simulink model "TotLabs_DCM"  (R2024b)
settings: Solver=VariableStepAuto  StartTime=0.0  StopTime=10.0  RelTol=1e-3
values from neighbouring files (symbols this model uses):
  Ar = [6e-2; 6e-2; 6e-2; 6e-2; 4e-2; 4e-2; 12e-2; 12e-2; 12e-2; 12e-2]    [LabsDCM.m]    (also in Srp_Lab7.m; airdrag.m)
  c = astroConstants(5)    [LabsDCM.m]    (also in Srp_Lab7.m; airdrag.m)
  Ep = deg2rad(epsilon)    [LabsDCM.m]    (also in Srp_Lab7.m = deg2rad(23.45); airdrag.m)
  Fe = 1358    [LabsDCM.m]    (also in airdrag.m)
  J = diag([Ix Iy Iz])    [LabsDCM.m]    (also in Srp_Lab7.m; airdrag.m)
  n = sqrt(G*M/(R^3))    [LabsDCM.m]    (also in Srp_Lab7.m; airdrag.m)
  N_B = [ 1,  0,  0 ... (first row only)    [LabsDCM.m]    (also in Srp_Lab7.m; airdrag.m)
  nx = 2*pi()/T    [LabsDCM.m]    (also in Srp_Lab7.m; airdrag.m)
  r_Fi = [ ... (first row only)    [LabsDCM.m]    (also in Srp_Lab7.m; airdrag.m)
  r_sun = astroConstants(2)    [LabsDCM.m]    (also in Srp_Lab7.m; airdrag.m = astroConstants(3))
  rho_d = [0.1; 0.1; 0.1; 0.1; 0.1; 0.1; 0.1; 0.1; 0.1; 0.1]    [LabsDCM.m]    (also in Srp_Lab7.m; airdrag.m)
  rho_s = [0.5; 0.5; 0.5; 0.5; 0.5; 0.5; 0.1; 0.1; 0.1; 0.1]    [LabsDCM.m]    (also in Srp_Lab7.m; airdrag.m)
  W0 = [0.45 0.52 0.55]    [LabsDCM.m]    (also in Srp_Lab7.m; airdrag.m)
libraries: matrix_library x3, vrlib x1
settings Model: Creator=User  LastModifiedBy=User

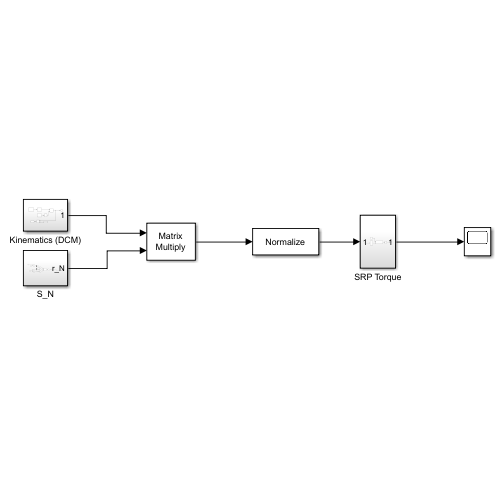
[thumbnail: Simulink's stored preview of the top-level diagram]
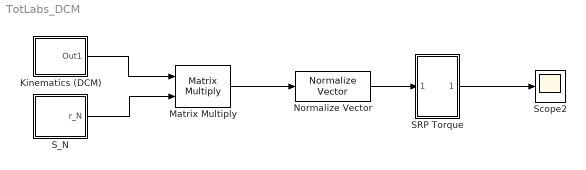
== system TotLabs_DCM ==
  Kinematics (DCM) : Subsystem
  Matrix Multiply : Product  Multiplication=Matrix(*)
  Normalize Vector : vrlib/Utilities/Normalize Vector  maxzero=0
  SRP Torque : Subsystem
  S_N : Subsystem
  Scope2 : Scope
  wires:
  Normalize Vector/1 -> SRP Torque/1(In1)
  SRP Torque/1(Out1) -> Scope2/1
  Matrix Multiply/1 -> Normalize Vector/1
  Kinematics (DCM)/1(Out1) -> Matrix Multiply/1
  S_N/1(r_N) -> Matrix Multiply/2

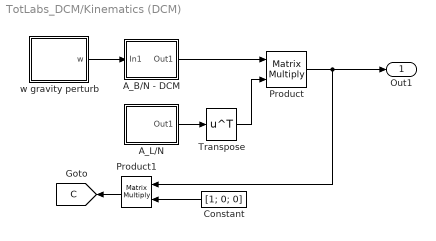
== system TotLabs_DCM/Kinematics (DCM) ==
  A_B/N - DCM : Subsystem
  A_L/N : Subsystem
  Constant : Constant  Value=[1; 0; 0]
  Product : Product  Multiplication=Matrix(*)
  Product1 : Product  Multiplication=Matrix(*)
  Transpose : Math  Operator=transpose
  w gravity perturb : Subsystem
  Out1 : Outport
  tag scope: C=global
  wires:
  A_L/N/1(Out1) -> Transpose/1
  Constant/1 -> Product1/2
  Product/1 -> Out1/1, Product1/1
  Transpose/1 -> Product/2
  A_B/N - DCM/1(Out1) -> Product/1
  Product1/1 -> [C]
  w gravity perturb/1(w) -> A_B/N - DCM/1(In1)

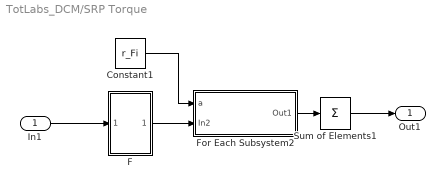
== system TotLabs_DCM/SRP Torque ==
  In1 : Inport
  Constant1 : Constant  Value=r_Fi
  F : Subsystem
  For Each Subsystem2 : Subsystem  TreatAsAtomicUnit=on
  Sum of Elements1 : Sum  Inputs=+  CollapseMode=Specified dimension
  Out1 : Outport
  wires:
  Constant1/1 -> For Each Subsystem2/1(a)
  For Each Subsystem2/1(Out1) -> Sum of Elements1/1
  Sum of Elements1/1 -> Out1/1
  In1/1 -> F/1(In1)
  F/1(Out1) -> For Each Subsystem2/2(In2)

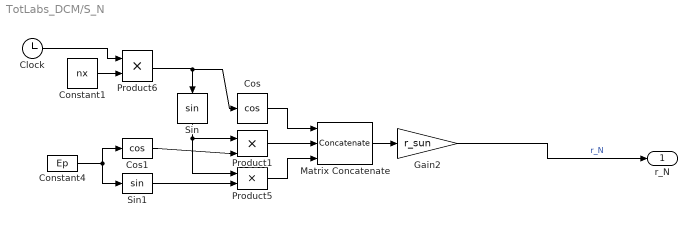
== system TotLabs_DCM/S_N ==
  Clock : Clock
  Constant1 : Constant  Value=nx
  Constant4 : Constant  Value=Ep
  Cos : Trigonometry  Operator=cos
  Cos1 : Trigonometry  Operator=cos
  Gain2 : Gain  Gain=r_sun
  Matrix Concatenate : Concatenate  NumInputs=3  Mode=Multidimensional array
  Product1 : Product
  Product5 : Product
  Product6 : Product
  Sin : Trigonometry
  Sin1 : Trigonometry
  r_N : Outport
  wires:
  Matrix Concatenate/1 -> Gain2/1
  Cos1/1 -> Product1/2
  Constant1/1 -> Product6/2
  Cos/1 -> Matrix Concatenate/1
  Product5/1 -> Matrix Concatenate/3
  Sin/1 -> Product5/1, Product1/1
  Clock/1 -> Product6/1
  Product1/1 -> Matrix Concatenate/2
  Sin1/1 -> Product5/2
  Product6/1 -> Cos/1, Sin/1
  Constant4/1 -> Sin1/1, Cos1/1
  Gain2/1 -> r_N/1  "r_N"

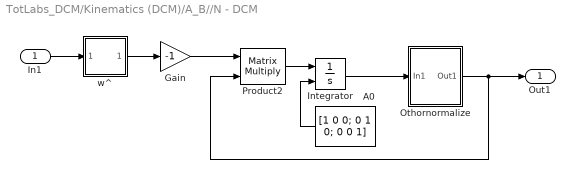
== system TotLabs_DCM/Kinematics (DCM)/A_B//N - DCM ==
  In1 : Inport
  A0 : Constant  Value=[1 0 0; 0 1 0; 0 0 1]
  Gain : Gain  Gain=-1
  Integrator : Integrator  InitialConditionSource=external
  Othornormalize : Subsystem
  Product2 : Product  Multiplication=Matrix(*)
  w^ : Subsystem
  Out1 : Outport
  wires:
  w^/1(Out1) -> Gain/1
  A0/1 -> Integrator/2
  Product2/1 -> Integrator/1
  In1/1 -> w^/1(In1)
  Othornormalize/1(Out1) -> Out1/1, Product2/2
  Integrator/1 -> Othornormalize/1(In1)
  Gain/1 -> Product2/1

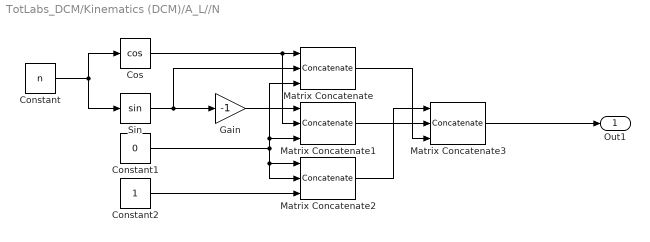
== system TotLabs_DCM/Kinematics (DCM)/A_L//N ==
  Constant : Constant  Value=n
  Constant1 : Constant  Value=0
  Constant2 : Constant
  Cos : Trigonometry  Operator=cos
  Gain : Gain  Gain=-1
  Matrix Concatenate : Concatenate  NumInputs=3  Mode=Multidimensional array
  Matrix Concatenate1 : Concatenate  NumInputs=3  Mode=Multidimensional array
  Matrix Concatenate2 : Concatenate  NumInputs=3  Mode=Multidimensional array
  Matrix Concatenate3 : Concatenate  NumInputs=3  Mode=Multidimensional array  ConcatenateDimension=2
  Sin : Trigonometry
  Out1 : Outport
  wires:
  Matrix Concatenate1/1 -> Matrix Concatenate3/2
  Matrix Concatenate3/1 -> Out1/1
  Constant1/1 -> Matrix Concatenate/3, Matrix Concatenate1/3, Matrix Concatenate2/2, Matrix Concatenate2/1
  Cos/1 -> Matrix Concatenate1/2, Matrix Concatenate/1
  Constant/1 -> Sin/1, Cos/1
  Constant2/1 -> Matrix Concatenate2/3
  Sin/1 -> Matrix Concatenate/2, Gain/1
  Gain/1 -> Matrix Concatenate1/1
  Matrix Concatenate2/1 -> Matrix Concatenate3/1
  Matrix Concatenate/1 -> Matrix Concatenate3/3

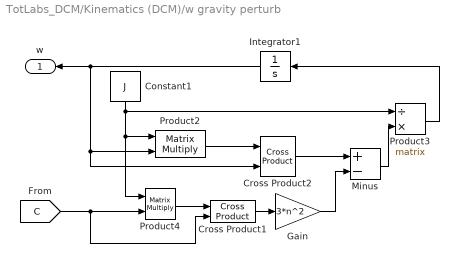
== system TotLabs_DCM/Kinematics (DCM)/w gravity perturb ==
  Constant1 : Constant  Value=J
  Cross Product1 : matrix_library/Cross Product
  Cross Product2 : matrix_library/Cross Product
  Gain : Gain  Gain=3*n^2
  Integrator1 : Integrator  InitialCondition=W0
  Minus : Sum  Inputs=+-
  Product2 : Product  Multiplication=Matrix(*)
  Product3 : Product  Inputs=/*  Multiplication=Matrix(*)
  Product4 : Product  Multiplication=Matrix(*)
  w : Outport
  wires:
  Integrator1/1 -> Cross Product2/2, Product2/2, w/1
  Minus/1 -> Product3/2
  Constant1/1 -> Product3/1, Product2/1, Product4/1
  Product3/1 -> Integrator1/1
  Product2/1 -> Cross Product2/1
  Cross Product2/1 -> Minus/1
  Cross Product1/1 -> Gain/1
  Gain/1 -> Minus/2
  Product4/1 -> Cross Product1/1
  [C] -> Product4/2, Cross Product1/2

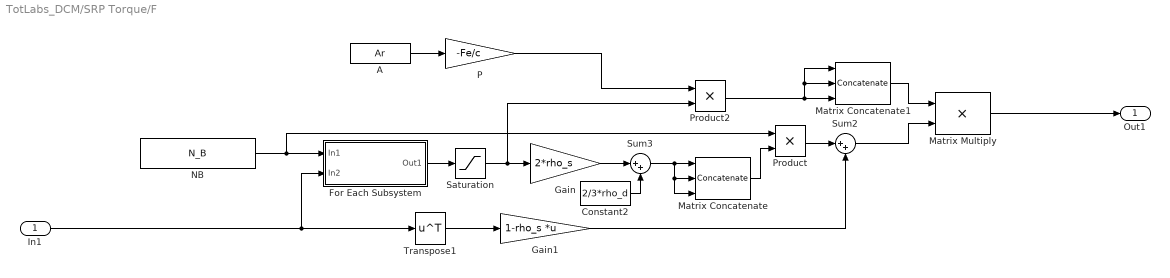
== system TotLabs_DCM/SRP Torque/F ==
  In1 : Inport
  A : Constant  Value=Ar
  Constant2 : Constant  Value=2/3*rho_d
  For Each Subsystem : Subsystem  TreatAsAtomicUnit=on
  Gain : Gain  Gain=2*rho_s
  Gain1 : Gain  Gain=1-rho_s  Multiplication=Matrix(K*u)
  Matrix Concatenate : Concatenate  NumInputs=3  Mode=Multidimensional array  ConcatenateDimension=2
  Matrix Concatenate1 : Concatenate  NumInputs=3  Mode=Multidimensional array  ConcatenateDimension=2
  Matrix Multiply : Product
  NB : Constant  Value=N_B
  P : Gain  Gain=-Fe/c
  Product : Product
  Product2 : Product
  Saturation : Saturate  UpperLimit=inf  LowerLimit=0
  Sum2 : Sum  Inputs=|++
  Sum3 : Sum  Inputs=|++
  Transpose1 : Math  Operator=transpose
  Out1 : Outport
  wires:
  For Each Subsystem/1(Out1) -> Saturation/1
  In1/1 -> For Each Subsystem/2(In2), Transpose1/1
  Matrix Concatenate/1 -> Product/2
  Gain/1 -> Sum3/1
  Saturation/1 -> Product2/2, Gain/1
  NB/1 -> For Each Subsystem/1(In1), Product/1
  Gain1/1 -> Sum2/2
  Matrix Concatenate1/1 -> Matrix Multiply/1
  Constant2/1 -> Sum3/2
  Sum3/1 -> Matrix Concatenate/1, Matrix Concatenate/3, Matrix Concatenate/2
  Product2/1 -> Matrix Concatenate1/3, Matrix Concatenate1/2, Matrix Concatenate1/1
  Product/1 -> Sum2/1
  P/1 -> Product2/1
  Sum2/1 -> Matrix Multiply/2
  Transpose1/1 -> Gain1/1
  A/1 -> P/1
  Matrix Multiply/1 -> Out1/1

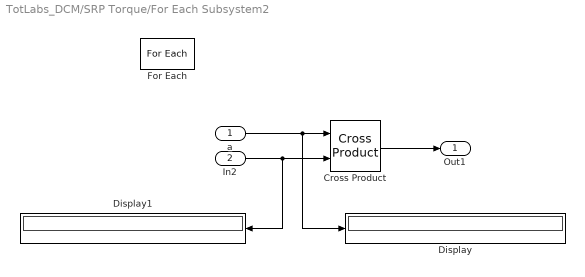
== system TotLabs_DCM/SRP Torque/For Each Subsystem2 ==
  a : Inport  Partition=on  PartitionDimension=1  PartitionWidth=1  PartitionOffset=0
  In2 : Inport  Port=2  Partition=on  PartitionDimension=1  PartitionWidth=1  PartitionOffset=0
  Cross Product : matrix_library/Cross Product
  Display : Display
  Display1 : Display
  For Each : ForEach  DisableCoverage=on
  Out1 : Outport  ConcatenationDimension=1
  wires:
  a/1 -> Display/1, Cross Product/1
  In2/1 -> Display1/1, Cross Product/2
  Cross Product/1 -> Out1/1

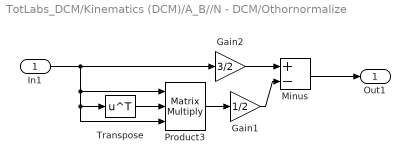
== system TotLabs_DCM/Kinematics (DCM)/A_B//N - DCM/Othornormalize ==
  In1 : Inport
  Gain1 : Gain  Gain=1/2
  Gain2 : Gain  Gain=3/2
  Minus : Sum  Inputs=+-
  Product3 : Product  Inputs=3  Multiplication=Matrix(*)
  Transpose : Math  Operator=transpose
  Out1 : Outport
  wires:
  Gain1/1 -> Minus/2
  Gain2/1 -> Minus/1
  In1/1 -> Product3/3, Transpose/1, Product3/1, Gain2/1
  Transpose/1 -> Product3/2
  Product3/1 -> Gain1/1
  Minus/1 -> Out1/1

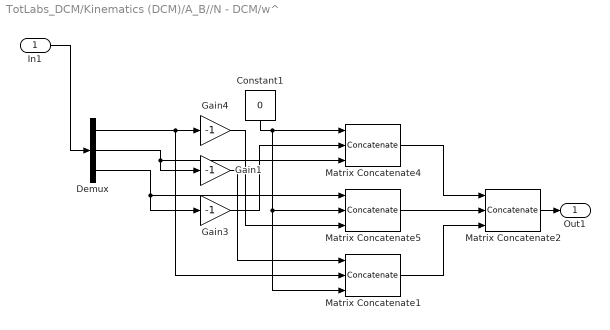
== system TotLabs_DCM/Kinematics (DCM)/A_B//N - DCM/w^ ==
  In1 : Inport
  Constant1 : Constant  Value=0
  Demux : Demux  Outputs=3
  Gain1 : Gain  Gain=-1
  Gain3 : Gain  Gain=-1
  Gain4 : Gain  Gain=-1
  Matrix Concatenate1 : Concatenate  NumInputs=3  Mode=Multidimensional array  ConcatenateDimension=2
  Matrix Concatenate2 : Concatenate  NumInputs=3  Mode=Multidimensional array
  Matrix Concatenate4 : Concatenate  NumInputs=3  Mode=Multidimensional array  ConcatenateDimension=2
  Matrix Concatenate5 : Concatenate  NumInputs=3  Mode=Multidimensional array  ConcatenateDimension=2
  Out1 : Outport
  wires:
  Matrix Concatenate1/1 -> Matrix Concatenate2/3
  Gain3/1 -> Matrix Concatenate4/2
  Constant1/1 -> Matrix Concatenate4/1, Matrix Concatenate5/2, Matrix Concatenate1/3
  Demux/3 -> Gain3/1, Matrix Concatenate5/1
  Demux/1 -> Gain4/1, Matrix Concatenate1/2
  Matrix Concatenate5/1 -> Matrix Concatenate2/2
  Demux/2 -> Gain1/1, Matrix Concatenate4/3
  Matrix Concatenate4/1 -> Matrix Concatenate2/1
  Gain4/1 -> Matrix Concatenate5/3
  Gain1/1 -> Matrix Concatenate1/1
  Matrix Concatenate2/1 -> Out1/1
  In1/1 -> Demux/1

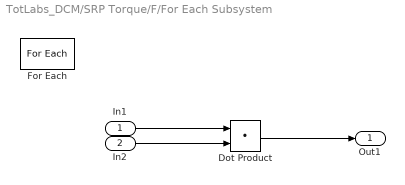
== system TotLabs_DCM/SRP Torque/F/For Each Subsystem ==
  In1 : Inport  Partition=on  PartitionDimension=1  PartitionWidth=1  PartitionOffset=0
  In2 : Inport  Port=2
  Dot Product : DotProduct  OutDataTypeStr=Inherit: Inherit via internal rule
  For Each : ForEach  DisableCoverage=on  SpecifiedNumIters=10
  Out1 : Outport  ConcatenationDimension=1
  wires:
  In1/1 -> Dot Product/1
  Dot Product/1 -> Out1/1
  In2/1 -> Dot Product/2
